simulink model "CP_ContrSys_Lin_a_n9464263_2019"  (R2019b)
settings: Solver=VariableStepAuto  StartTime=0.0  StopTime=10.0  RelTol=1e-3
values from neighbouring files (symbols this model uses):
  A = double(subs(B_jac, x_bar, fixed_point))    [nonlinear_dynamics.m]
  B = double(subs(A_jac, x_bar, fixed_point))    [nonlinear_dynamics.m]
  C = [1 0 0 0 ... (first row only)    [nonlinear_dynamics.m]
  D = 0    [nonlinear_dynamics.m]
  K = place(A, B, [-3, -4, -5, -6])    [nonlinear_dynamics.m]
  L = place(A', C', [-63, -64, -65, -66])'    [nonlinear_dynamics.m]
  x0 = [0.2 20*pi/180 0 0]'    [CP_ContrSys_a_MainFile_n9464263.m]    (also in CP_ContrSys_b_MainFile_n9464263.m = [0.2 200*pi/180 0 0]'; nonlinear_dynamics.m = [0 0 0 0]')
  x_bar = x_bar_a    [CP_ContrSys_a_MainFile_n9464263.m]    (also in CP_ContrSys_b_MainFile_n9464263.m = x_bar_b; nonlinear_dynamics.m = sym('x_bar_', [4, 1]))
settings Model: Creator=cal  LastModifiedBy=cal

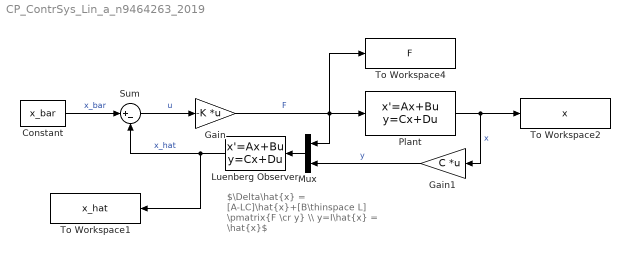
== system CP_ContrSys_Lin_a_n9464263_2019 ==
  note: $\Delta\hat{x} = [A-LC]\hat{x}+[B\thinspace L] \pmatrix{F \cr y} \\ y=I\hat{x} = \hat{x}$
  Constant : Constant  Value=x_bar
  Gain : Gain  Gain=-K  Multiplication=Matrix(K*u)
  Gain1 : Gain  Gain=C  Multiplication=Matrix(K*u)
  Luenberg Observer : StateSpace  A=A - L * C  B=[B L]  C=eye(size(A))  D=zeros(size([B L])) % TODO: handle nonzero D  InitialCondition=x0
  Mux : Mux  Inputs=2
  Plant : StateSpace  A=A  B=B  C=eye(size(A))  D=zeros(size(B))  InitialCondition=x0
  Sum : Sum  Inputs=|+-
  To Workspace1 : ToWorkspace  VariableName=x_hat  SampleTime=-1
  To Workspace2 : ToWorkspace  VariableName=x  SampleTime=-1
  To Workspace4 : ToWorkspace  VariableName=F  SampleTime=-1
  wires:
  Sum/1 -> Gain/1  "u"
  Plant/1 -> Gain1/1, To Workspace2/1  "x"
  Mux/1 -> Luenberg Observer/1
  Luenberg Observer/1 -> To Workspace1/1, Sum/2  "x_hat"
  Constant/1 -> Sum/1  "x_bar"
  Gain1/1 -> Mux/2  "y"
  Gain/1 -> Mux/1, To Workspace4/1, Plant/1  "F"
